simulink model "non_fuzzy_weights"  (Simulink 8.2)
settings: Solver=ode45  StartTime=0.0  StopTime=10.0  RelTol=1e-3
settings Model: Creator=ali  LastModifiedBy=ali
settings DataIOCC: SignalLoggingSaveFormat=Dataset
settings OptimizationCC: ExpressionDepthLimit=128
settings DebuggingCC: FcnCallInpInsideContextMsg=EnableAllAsError  StateNameClashWarn=none
settings GRTTargetCC: CombineOutputUpdateFcns=on  GRTInterface=off

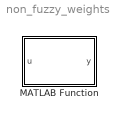
== system non_fuzzy_weights ==
  MATLAB Function : MATLAB Function  TreatAsAtomicUnit=on

== matlab function MATLAB Function ==
  data: u input double; y output double
function y = fcn(u)
inp = u;
[val_max,num_max]=max(inp);
y=u;
for i=1:4
    if i==num_max
        y(i)=1;
    else
        y(i)=0;
    end
end
